simulink library "sm_boom_lift_crawler_lib"  (R2026a)
settings: Solver=VariableStepAuto
undefined symbols (not defined in the file): B, b, base_clr_a, base_clr_d, base_clr_e, base_clr_h, base_clr_s, base_h, base_opc, base_rho, base_t, base_w, F, lines, motion, overlap_l, valves, X, Y, Z
libraries: nesl_utility x155, fl_lib x72, sm_lib x38, SimscapeFluids_lib x18, $bdroot x2, simulink_extras x1, simulink x1, Custom_Valves x1
(part 1 of 4)
Description:
  | Copyright 2020-2026 The MathWorks, Inc.
settings Model: Creator=smiller  LastModifiedBy=smiller

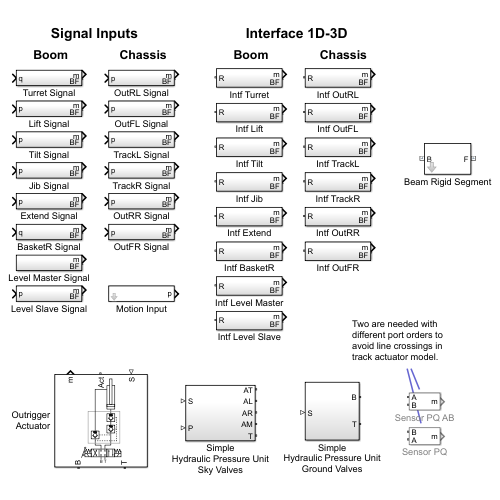
[thumbnail: Simulink's stored preview of the top-level diagram]
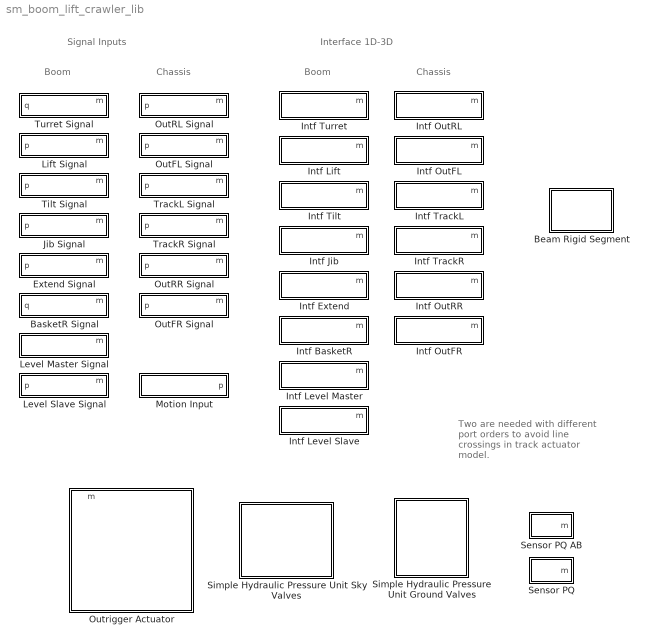
== system sm_boom_lift_crawler_lib ==
  note: Two are needed with different port orders to avoid line crossings in track actuator model.
  note: Boom
  note: Interface 1D-3D
  note: Chassis
  note: Boom
  note: Signal Inputs
  note: Chassis
  BasketR Signal : Subsystem
  Beam Rigid Segment : Subsystem  mask{beam_h=base_h, beam_w=base_w, beam_t=base_t, beam_l=overlap_l, beam_rho=base_rho, clr_d=base_clr_d, clr_s=base_clr_s, clr_a=base_clr_a, clr_e=base_clr_e, clr_h=base_clr_h, opc=base_opc}
      mask prompts: beam_h "Height (ft)"; beam_w "Width (ft)"; beam_t "Thickness (ft)"; beam_l "Length (ft)"; beam_rho "Density (kg/m^3)"; clr_d "Diffuse Color"; clr_s "Specular Color"; clr_a "Ambient Color"; clr_e "Emissive Color"; clr_h "Shininess"; opc "Opacity (0-1)"
      mask init:
      | beam_extr = [...
      |      beam_w/2  beam_h/2;
      |     -beam_w/2  beam_h/2;
      |     -beam_w/2 -beam_h/2;
      |      beam_w/2 -beam_h/2;
      |      beam_w/2  beam_h/2;
      |      (beam_w/2-beam_t)  (beam_h/2-beam_t);
      |      (beam_w/2-beam_t) -(beam_h/2-beam_t);
      |     -(beam_w/2-beam_t) -(beam_h/2-beam_t);
      |     -(beam_w/2-beam_t)  (beam_h/2-beam_t);
      |      (beam_w/2-beam_t)  (beam_h/2-beam_t);
      |     ];
      mask DialogControl cont_vis Prompt: Visualization
  Extend Signal : Subsystem
  Intf BasketR : Subsystem
  Intf Extend : Subsystem
  Intf Jib : Subsystem
  Intf Level Master : Subsystem
  Intf Level Slave : Subsystem
  Intf Lift : Subsystem
  Intf OutFL : Subsystem
  Intf OutFR : Subsystem
  Intf OutRL : Subsystem
  Intf OutRR : Subsystem
  Intf Tilt : Subsystem
  Intf TrackL : Subsystem
  Intf TrackR : Subsystem
  Intf Turret : Subsystem
  Jib Signal : Subsystem
  Level Master Signal : Subsystem
  Level Slave Signal : Subsystem
  Lift Signal : Subsystem
  Motion Input : Subsystem  mask{vec_t=motion.turret.t, vec_q=motion.turret.q}
      mask prompts: vec_t "Time"; vec_q "Angles (rad)"
  OutFL Signal : Subsystem
  OutFR Signal : Subsystem
  OutRL Signal : Subsystem
  OutRR Signal : Subsystem
  Outrigger Actuator : Subsystem
      mask Display: image('sh009.svg')
  Sensor PQ : Subsystem
  Sensor PQ AB : Subsystem
  Simple Hydraulic Pressure Unit Ground Valves : Subsystem
  Simple Hydraulic Pressure Unit Sky Valves : Subsystem
  Tilt Signal : Subsystem
  TrackL Signal : Subsystem
  TrackR Signal : Subsystem
  Turret Signal : Subsystem

== system sm_boom_lift_crawler_lib/BasketR Signal ==
  q : Inport
  Bus Creator1 : BusCreator  Inputs=3
  PS-Simulink Converter1 : nesl_utility/PS-Simulink Converter  PhysicalDomain=network_engine_domain  SubClassName=ps_output  LeftPortType=input  RightPortType=output  PseudoPeriodic=off  Frequencies=[]  VectorFormat=1-D array  Unit=inherit  AffineConversion=off
  PS-Simulink Converter2 : nesl_utility/PS-Simulink Converter  PhysicalDomain=network_engine_domain  SubClassName=ps_output  LeftPortType=input  RightPortType=output  PseudoPeriodic=off  Frequencies=[]  VectorFormat=1-D array  Unit=inherit  AffineConversion=off
  PS-Simulink Converter3 : nesl_utility/PS-Simulink Converter  PhysicalDomain=network_engine_domain  SubClassName=ps_output  LeftPortType=input  RightPortType=output  PseudoPeriodic=off  Frequencies=[]  VectorFormat=1-D array  Unit=inherit  AffineConversion=off
  Revolute BasketR : sm_lib/Joints/Revolute Joint  JointMode=Normal  CompositeWrenchDir=FollowerOnBase  CompositeWrenchFrame=BaseFrame  SenseConstraintForce=off  SenseConstraintTorque=off  SenseTotalForce=off  SenseTotalTorque=off  PositionTargetSpecify=on  PositionTargetPriority=High  PositionTargetValue=0  PositionTargetValueUnits=deg  VelocityTargetSpecify=off  VelocityTargetPriority=High  VelocityTargetValue=0  VelocityTargetValueUnits=deg/s  EquilibriumPosition=0  EquilibriumPositionUnits=rad  SpringStiffness=0  SpringStiffnessUnits=N*m/rad  DampingCoefficient=b.r.joint  DampingCoefficientUnits=N*m/(rad/s)  LowerLimitSpecify=on  LowerLimitBound=-180  LowerLimitBoundUnits=deg  LowerLimitStiffness=1e4  LowerLimitStiffnessUnits=N*m/deg  LowerLimitDamping=10  LowerLimitDampingUnits=N*m/(deg/s)  LowerLimitTransitionRegionWidth=0.1  LowerLimitTransitionRegionWidthUnits=deg  UpperLimitSpecify=on  UpperLimitBound=180  UpperLimitBoundUnits=deg  UpperLimitStiffness=1e4  UpperLimitStiffnessUnits=N*m/deg  UpperLimitDamping=10  UpperLimitDampingUnits=N*m/(deg/s)  UpperLimitTransitionRegionWidth=0.1  UpperLimitTransitionRegionWidthUnits=deg  TorqueActuationMode=ComputedTorque  MotionActuationMode=InputMotion  SensePosition=on  SenseVelocity=on  SenseAcceleration=off  SenseTorqueForce=on  SenseLowerLimitTorqueForce=off  SenseUpperLimitTorqueForce=off
  Simscape Bus3 : SimscapeBus  HierarchyStrings=B;F
  Simulink-PS Converter : nesl_utility/Simulink-PS Converter  PhysicalDomain=network_engine_domain  SubClassName=ps_input  LeftPortType=input  RightPortType=output  PseudoPeriodic=off  Frequencies=[]  NoiseDistribution=none  NoiseParameters=[]  Unit=rad  AffineConversion=off  FilteringAndDerivatives=filter  SimscapeFilterOrder=2  InputFilterTimeConstant=0.1  UdotUserProvided=0
  BF : PMIOPort  Side=Right
  m : Outport
  wires:
  PS-Simulink Converter3/1 -> Bus Creator1/3  "t"
  PS-Simulink Converter1/1 -> Bus Creator1/1  "q"
  PS-Simulink Converter2/1 -> Bus Creator1/2  "w"
  Bus Creator1/1 -> m/1  "BasketR"
  q/1 -> Simulink-PS Converter/1
  connections:
  PS-Simulink Converter3/LConn1 -- Revolute BasketR/RConn4
  Revolute BasketR/LConn2 -- Simulink-PS Converter/RConn1
  Simscape Bus3/LConn1 -- Revolute BasketR/LConn1
  Revolute BasketR/RConn3 -- PS-Simulink Converter2/LConn1
  Simscape Bus3/LConn2 -- Revolute BasketR/RConn1
  PS-Simulink Converter1/LConn1 -- Revolute BasketR/RConn2
  Simscape Bus3/RConn1 -- BF/RConn1

== system sm_boom_lift_crawler_lib/Beam Rigid Segment ==
  Bottom : sm_lib/Body Elements/Brick Solid  BrickDimensions=[beam_w beam_t overlap_l]  BrickDimensionsUnits=ft  ExportEntireGeometry=off  InertiaType=CalculateFromGeometry  BasedOnType=Density  Density=beam_rho  DensityUnits=kg/m^3  Mass=1  MassUnits=kg  CenterOfMass=[0 0 0]  CenterOfMassUnits=m  MomentsOfInertia=[1 1 1]  MomentsOfInertiaUnits=kg*m^2  ProductsOfInertia=[0 0 0]  ProductsOfInertiaUnits=kg*m^2  GraphicType=FromGeometry  MarkerShape=Sphere  MarkerSize=10  GraphicVisPropType=SimpleVisualProperties  GraphicDiffuseColor=clr_d  GraphicOpacity=opc  GraphicSpecularColor=clr_s  GraphicAmbientColor=clr_a  GraphicEmissiveColor=clr_e  GraphicShininess=clr_h  DoExposeReferenceFrame=on  SerializedFrames=<Frames/>
  Left : sm_lib/Body Elements/Brick Solid  BrickDimensions=[beam_t beam_h-beam_t*2 overlap_l]  BrickDimensionsUnits=ft  ExportEntireGeometry=off  InertiaType=CalculateFromGeometry  BasedOnType=Density  Density=beam_rho  DensityUnits=kg/m^3  Mass=1  MassUnits=kg  CenterOfMass=[0 0 0]  CenterOfMassUnits=m  MomentsOfInertia=[1 1 1]  MomentsOfInertiaUnits=kg*m^2  ProductsOfInertia=[0 0 0]  ProductsOfInertiaUnits=kg*m^2  GraphicType=FromGeometry  MarkerShape=Sphere  MarkerSize=10  GraphicVisPropType=SimpleVisualProperties  GraphicDiffuseColor=clr_d  GraphicOpacity=opc  GraphicSpecularColor=clr_s  GraphicAmbientColor=clr_a  GraphicEmissiveColor=clr_e  GraphicShininess=clr_h  DoExposeReferenceFrame=on  SerializedFrames=<Frames/>
  Right : sm_lib/Body Elements/Brick Solid  BrickDimensions=[beam_t beam_h-beam_t*2 overlap_l]  BrickDimensionsUnits=ft  ExportEntireGeometry=off  InertiaType=CalculateFromGeometry  BasedOnType=Density  Density=beam_rho  DensityUnits=kg/m^3  Mass=1  MassUnits=kg  CenterOfMass=[0 0 0]  CenterOfMassUnits=m  MomentsOfInertia=[1 1 1]  MomentsOfInertiaUnits=kg*m^2  ProductsOfInertia=[0 0 0]  ProductsOfInertiaUnits=kg*m^2  GraphicType=FromGeometry  MarkerShape=Sphere  MarkerSize=10  GraphicVisPropType=SimpleVisualProperties  GraphicDiffuseColor=clr_d  GraphicOpacity=opc  GraphicSpecularColor=clr_s  GraphicAmbientColor=clr_a  GraphicEmissiveColor=clr_e  GraphicShininess=clr_h  DoExposeReferenceFrame=on  SerializedFrames=<Frames/>
  Top : sm_lib/Body Elements/Brick Solid  BrickDimensions=[beam_w beam_t overlap_l]  BrickDimensionsUnits=ft  ExportEntireGeometry=off  InertiaType=CalculateFromGeometry  BasedOnType=Density  Density=beam_rho  DensityUnits=kg/m^3  Mass=1  MassUnits=kg  CenterOfMass=[0 0 0]  CenterOfMassUnits=m  MomentsOfInertia=[1 1 1]  MomentsOfInertiaUnits=kg*m^2  ProductsOfInertia=[0 0 0]  ProductsOfInertiaUnits=kg*m^2  GraphicType=FromGeometry  MarkerShape=Sphere  MarkerSize=10  GraphicVisPropType=SimpleVisualProperties  GraphicDiffuseColor=clr_d  GraphicOpacity=opc  GraphicSpecularColor=clr_s  GraphicAmbientColor=clr_a  GraphicEmissiveColor=clr_e  GraphicShininess=clr_h  DoExposeReferenceFrame=on  SerializedFrames=<Frames/>
  Transform B Center : sm_lib/Frames and Transforms/Rigid Transform  RotationMethod=None  FollAlignAxisA=+X  BaseAlignAxisA=+Y  FollAlignAxisB=+Y  BaseAlignAxisB=+Z  RotationStandardAxis=+Z  RotationAngle=0.0  RotationAngleUnits=deg  RotationArbitraryAxis=[0 0 1]  RotationSequenceAxes=FollowerAxes  RotationSequence=XYX  RotationSequenceAngles=[0 0 0]  RotationSequenceAnglesUnits=deg  RotationMatrix=[1 0 0; 0 1 0; 0 0 1]  Quaternion=[1 0 0 0]  TranslationMethod=StandardAxis  TranslationCartesianOffset=[0 0 0]  TranslationCartesianOffsetUnits=ft  TranslationStandardAxis=+Z  TranslationStandardOffset=overlap_l/2  TranslationStandardOffsetUnits=ft  TranslationROffset=0  TranslationROffsetUnits=m  TranslationThetaOffset=0  TranslationThetaOffsetUnits=deg  TranslationZOffset=0  TranslationZOffsetUnits=m
  Transform Bottom : sm_lib/Frames and Transforms/Rigid Transform  RotationMethod=None  FollAlignAxisA=+X  BaseAlignAxisA=+Y  FollAlignAxisB=+Y  BaseAlignAxisB=+Z  RotationStandardAxis=+Y  RotationAngle=0.0  RotationAngleUnits=deg  RotationArbitraryAxis=[0 0 1]  RotationSequenceAxes=FollowerAxes  RotationSequence=XYX  RotationSequenceAngles=[0 0 0]  RotationSequenceAnglesUnits=deg  RotationMatrix=[1 0 0; 0 1 0; 0 0 1]  Quaternion=[1 0 0 0]  TranslationMethod=StandardAxis  TranslationCartesianOffset=[0 0 0]  TranslationCartesianOffsetUnits=ft  TranslationStandardAxis=+Y  TranslationStandardOffset=(beam_h-beam_t)/2  TranslationStandardOffsetUnits=ft  TranslationROffset=0  TranslationROffsetUnits=m  TranslationThetaOffset=0  TranslationThetaOffsetUnits=deg  TranslationZOffset=0  TranslationZOffsetUnits=m
  Transform Center F : sm_lib/Frames and Transforms/Rigid Transform  RotationMethod=None  FollAlignAxisA=+X  BaseAlignAxisA=+Y  FollAlignAxisB=+Y  BaseAlignAxisB=+Z  RotationStandardAxis=+Z  RotationAngle=0.0  RotationAngleUnits=deg  RotationArbitraryAxis=[0 0 1]  RotationSequenceAxes=FollowerAxes  RotationSequence=XYX  RotationSequenceAngles=[0 0 0]  RotationSequenceAnglesUnits=deg  RotationMatrix=[1 0 0; 0 1 0; 0 0 1]  Quaternion=[1 0 0 0]  TranslationMethod=StandardAxis  TranslationCartesianOffset=[0 0 0]  TranslationCartesianOffsetUnits=ft  TranslationStandardAxis=+Z  TranslationStandardOffset=overlap_l/2  TranslationStandardOffsetUnits=ft  TranslationROffset=0  TranslationROffsetUnits=m  TranslationThetaOffset=0  TranslationThetaOffsetUnits=deg  TranslationZOffset=0  TranslationZOffsetUnits=m
  Transform Left : sm_lib/Frames and Transforms/Rigid Transform  RotationMethod=None  FollAlignAxisA=+X  BaseAlignAxisA=+Y  FollAlignAxisB=+Y  BaseAlignAxisB=+Z  RotationStandardAxis=+Y  RotationAngle=0.0  RotationAngleUnits=deg  RotationArbitraryAxis=[0 0 1]  RotationSequenceAxes=FollowerAxes  RotationSequence=XYX  RotationSequenceAngles=[0 0 0]  RotationSequenceAnglesUnits=deg  RotationMatrix=[1 0 0; 0 1 0; 0 0 1]  Quaternion=[1 0 0 0]  TranslationMethod=StandardAxis  TranslationCartesianOffset=[0 0 0]  TranslationCartesianOffsetUnits=ft  TranslationStandardAxis=+X  TranslationStandardOffset=(beam_w-beam_t)/2  TranslationStandardOffsetUnits=ft  TranslationROffset=0  TranslationROffsetUnits=m  TranslationThetaOffset=0  TranslationThetaOffsetUnits=deg  TranslationZOffset=0  TranslationZOffsetUnits=m
  Transform Right : sm_lib/Frames and Transforms/Rigid Transform  RotationMethod=None  FollAlignAxisA=+X  BaseAlignAxisA=+Y  FollAlignAxisB=+Y  BaseAlignAxisB=+Z  RotationStandardAxis=+Y  RotationAngle=0.0  RotationAngleUnits=deg  RotationArbitraryAxis=[0 0 1]  RotationSequenceAxes=FollowerAxes  RotationSequence=XYX  RotationSequenceAngles=[0 0 0]  RotationSequenceAnglesUnits=deg  RotationMatrix=[1 0 0; 0 1 0; 0 0 1]  Quaternion=[1 0 0 0]  TranslationMethod=StandardAxis  TranslationCartesianOffset=[0 0 0]  TranslationCartesianOffsetUnits=ft  TranslationStandardAxis=+X  TranslationStandardOffset=(beam_w-beam_t)/2  TranslationStandardOffsetUnits=ft  TranslationROffset=0  TranslationROffsetUnits=m  TranslationThetaOffset=0  TranslationThetaOffsetUnits=deg  TranslationZOffset=0  TranslationZOffsetUnits=m
  Transform Top : sm_lib/Frames and Transforms/Rigid Transform  RotationMethod=None  FollAlignAxisA=+X  BaseAlignAxisA=+Y  FollAlignAxisB=+Y  BaseAlignAxisB=+Z  RotationStandardAxis=+Y  RotationAngle=0.0  RotationAngleUnits=deg  RotationArbitraryAxis=[0 0 1]  RotationSequenceAxes=FollowerAxes  RotationSequence=XYX  RotationSequenceAngles=[0 0 0]  RotationSequenceAnglesUnits=deg  RotationMatrix=[1 0 0; 0 1 0; 0 0 1]  Quaternion=[1 0 0 0]  TranslationMethod=StandardAxis  TranslationCartesianOffset=[0 0 0]  TranslationCartesianOffsetUnits=ft  TranslationStandardAxis=+Y  TranslationStandardOffset=(beam_h-beam_t)/2  TranslationStandardOffsetUnits=ft  TranslationROffset=0  TranslationROffsetUnits=m  TranslationThetaOffset=0  TranslationThetaOffsetUnits=deg  TranslationZOffset=0  TranslationZOffsetUnits=m
  B : PMIOPort  Side=Left
  F : PMIOPort  Port=2  Side=Right
  connections:
  Left/RConn1 -- Transform Left/LConn1
  Right/RConn1 -- Transform Right/RConn1
  Bottom/RConn1 -- Transform Bottom/LConn1
  Top/RConn1 -- Transform Top/RConn1
  Transform Left/RConn1 -- Transform Top/LConn1 -- Transform Right/LConn1 -- Transform B Center/RConn1 -- Transform Center F/LConn1 -- Transform Bottom/RConn1
  Transform Center F/RConn1 -- F/RConn1
  Transform B Center/LConn1 -- B/RConn1

== system sm_boom_lift_crawler_lib/Extend Signal ==
  p : Inport
  Bus Creator1 : BusCreator  Inputs=3
  PS-Simulink Converter1 : nesl_utility/PS-Simulink Converter  PhysicalDomain=network_engine_domain  SubClassName=ps_output  LeftPortType=input  RightPortType=output  PseudoPeriodic=off  Frequencies=[]  VectorFormat=1-D array  Unit=inherit  AffineConversion=off
  PS-Simulink Converter2 : nesl_utility/PS-Simulink Converter  PhysicalDomain=network_engine_domain  SubClassName=ps_output  LeftPortType=input  RightPortType=output  PseudoPeriodic=off  Frequencies=[]  VectorFormat=1-D array  Unit=inherit  AffineConversion=off
  PS-Simulink Converter3 : nesl_utility/PS-Simulink Converter  PhysicalDomain=network_engine_domain  SubClassName=ps_output  LeftPortType=input  RightPortType=output  PseudoPeriodic=off  Frequencies=[]  VectorFormat=1-D array  Unit=inherit  AffineConversion=off
  Prismatic Extend : sm_lib/Joints/Prismatic Joint  JointMode=Normal  CompositeWrenchDir=FollowerOnBase  CompositeWrenchFrame=BaseFrame  SenseConstraintForce=off  SenseConstraintTorque=off  SenseTotalForce=off  SenseTotalTorque=off  PositionTargetSpecify=on  PositionTargetPriority=High  PositionTargetValue=pz0.stickboom.extend  PositionTargetValueUnits=in  VelocityTargetSpecify=off  VelocityTargetPriority=High  VelocityTargetValue=0  VelocityTargetValueUnits=m/s  EquilibriumPosition=0  EquilibriumPositionUnits=m  SpringStiffness=0  SpringStiffnessUnits=N/m  DampingCoefficient=0  DampingCoefficientUnits=N/(m/s)  LowerLimitSpecify=off  LowerLimitBound=0.125  LowerLimitBoundUnits=in  LowerLimitStiffness=1e6  LowerLimitStiffnessUnits=N/m  LowerLimitDamping=1e3  LowerLimitDampingUnits=N/(m/s)  LowerLimitTransitionRegionWidth=1e-4  LowerLimitTransitionRegionWidthUnits=m  UpperLimitSpecify=off  UpperLimitBound=170  UpperLimitBoundUnits=in  UpperLimitStiffness=1e6  UpperLimitStiffnessUnits=N/m  UpperLimitDamping=1e3  UpperLimitDampingUnits=N/(m/s)  UpperLimitTransitionRegionWidth=1e-4  UpperLimitTransitionRegionWidthUnits=m  TorqueActuationMode=ComputedTorque  MotionActuationMode=InputMotion  SensePosition=on  SenseVelocity=on  SenseAcceleration=off  SenseTorqueForce=on  SenseLowerLimitTorqueForce=off  SenseUpperLimitTorqueForce=off
  Simscape Bus3 : SimscapeBus  HierarchyStrings=B;F
  Simulink-PS Converter : nesl_utility/Simulink-PS Converter  PhysicalDomain=network_engine_domain  SubClassName=ps_input  LeftPortType=input  RightPortType=output  PseudoPeriodic=off  Frequencies=[]  NoiseDistribution=none  NoiseParameters=[]  Unit=m  AffineConversion=off  FilteringAndDerivatives=filter  SimscapeFilterOrder=2  InputFilterTimeConstant=0.2  UdotUserProvided=0
  BF : PMIOPort  Side=Right
  m : Outport
  wires:
  PS-Simulink Converter3/1 -> Bus Creator1/3  "f"
  Bus Creator1/1 -> m/1  "Extend"
  PS-Simulink Converter2/1 -> Bus Creator1/2  "v"
  p/1 -> Simulink-PS Converter/1
  PS-Simulink Converter1/1 -> Bus Creator1/1  "p"
  connections:
  PS-Simulink Converter3/LConn1 -- Prismatic Extend/RConn4
  PS-Simulink Converter2/LConn1 -- Prismatic Extend/RConn3
  Prismatic Extend/LConn2 -- Simulink-PS Converter/RConn1
  BF/RConn1 -- Simscape Bus3/RConn1
  Simscape Bus3/LConn1 -- Prismatic Extend/LConn1
  Prismatic Extend/RConn1 -- Simscape Bus3/LConn2
  PS-Simulink Converter1/LConn1 -- Prismatic Extend/RConn2

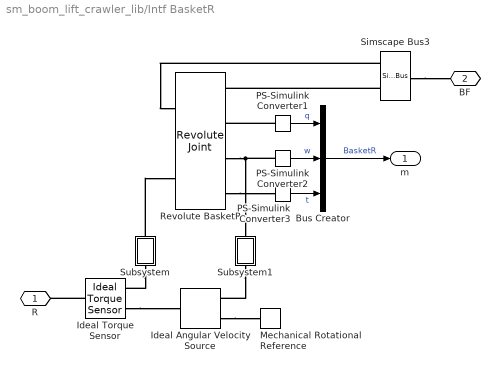
== system sm_boom_lift_crawler_lib/Intf BasketR ==
  Bus Creator : BusCreator  Inputs=3
  Ideal Angular Velocity Source : fl_lib/Mechanical/Mechanical Sources/Ideal Angular Velocity Source
  Ideal Torque Sensor : fl_lib/Mechanical/Mechanical Sensors/Ideal Torque Sensor
  Mechanical Rotational Reference : fl_lib/Mechanical/Rotational Elements/Mechanical Rotational Reference
  PS-Simulink Converter1 : nesl_utility/PS-Simulink Converter  PhysicalDomain=network_engine_domain  SubClassName=ps_output  LeftPortType=input  RightPortType=output  PseudoPeriodic=off  Frequencies=[]  VectorFormat=1-D array  Unit=inherit  AffineConversion=off
  PS-Simulink Converter2 : nesl_utility/PS-Simulink Converter  PhysicalDomain=network_engine_domain  SubClassName=ps_output  LeftPortType=input  RightPortType=output  PseudoPeriodic=off  Frequencies=[]  VectorFormat=1-D array  Unit=inherit  AffineConversion=off
  PS-Simulink Converter3 : nesl_utility/PS-Simulink Converter  PhysicalDomain=network_engine_domain  SubClassName=ps_output  LeftPortType=input  RightPortType=output  PseudoPeriodic=off  Frequencies=[]  VectorFormat=1-D array  Unit=inherit  AffineConversion=off
  Revolute BasketR : sm_lib/Joints/Revolute Joint  JointMode=Normal  CompositeWrenchDir=FollowerOnBase  CompositeWrenchFrame=BaseFrame  SenseConstraintForce=off  SenseConstraintTorque=off  SenseTotalForce=off  SenseTotalTorque=off  PositionTargetSpecify=on  PositionTargetPriority=High  PositionTargetValue=0  PositionTargetValueUnits=deg  VelocityTargetSpecify=off  VelocityTargetPriority=High  VelocityTargetValue=0  VelocityTargetValueUnits=deg/s  EquilibriumPosition=0  EquilibriumPositionUnits=rad  SpringStiffness=0  SpringStiffnessUnits=N*m/rad  DampingCoefficient=b.r.joint  DampingCoefficientUnits=N*m/(rad/s)  LowerLimitSpecify=on  LowerLimitBound=-180  LowerLimitBoundUnits=deg  LowerLimitStiffness=1e4  LowerLimitStiffnessUnits=N*m/deg  LowerLimitDamping=10  LowerLimitDampingUnits=N*m/(deg/s)  LowerLimitTransitionRegionWidth=0.1  LowerLimitTransitionRegionWidthUnits=deg  UpperLimitSpecify=on  UpperLimitBound=180  UpperLimitBoundUnits=deg  UpperLimitStiffness=1e4  UpperLimitStiffnessUnits=N*m/deg  UpperLimitDamping=10  UpperLimitDampingUnits=N*m/(deg/s)  UpperLimitTransitionRegionWidth=0.1  UpperLimitTransitionRegionWidthUnits=deg  TorqueActuationMode=InputTorque  MotionActuationMode=ComputedMotion  SensePosition=on  SenseVelocity=on  SenseAcceleration=off  SenseTorqueForce=on  SenseLowerLimitTorqueForce=off  SenseUpperLimitTorqueForce=off
  Simscape Bus3 : SimscapeBus  HierarchyStrings=B;F
  Subsystem : Subsystem
  Subsystem1 : Subsystem
  R : PMIOPort  Side=Left
  BF : PMIOPort  Port=2  Side=Right
  m : Outport
  wires:
  PS-Simulink Converter1/1 -> Bus Creator/1  "q"
  Bus Creator/1 -> m/1  "BasketR"
  PS-Simulink Converter2/1 -> Bus Creator/2  "w"
  PS-Simulink Converter3/1 -> Bus Creator/3  "t"
  connections:
  Simscape Bus3/LConn1 -- Revolute BasketR/LConn1
  Revolute BasketR/RConn3 -- Subsystem1/LConn1 -- PS-Simulink Converter2/LConn1
  Subsystem/RConn1 -- Revolute BasketR/LConn2
  Ideal Torque Sensor/LConn1 -- R/RConn1
  Simscape Bus3/LConn2 -- Revolute BasketR/RConn1
  PS-Simulink Converter1/LConn1 -- Revolute BasketR/RConn2
  Simscape Bus3/RConn1 -- BF/RConn1
  Subsystem1/RConn1 -- Ideal Angular Velocity Source/RConn1
  Ideal Angular Velocity Source/RConn2 -- Mechanical Rotational Reference/LConn1
  Ideal Torque Sensor/RConn1 -- Ideal Angular Velocity Source/LConn1
  Subsystem/LConn1 -- Ideal Torque Sensor/RConn2
  Revolute BasketR/RConn4 -- PS-Simulink Converter3/LConn1

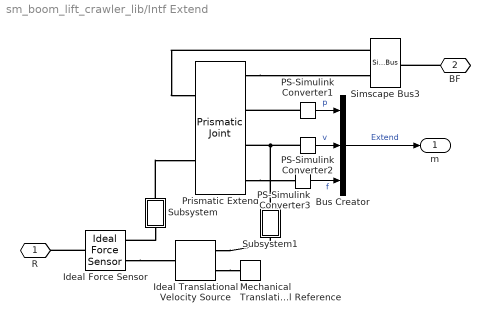
== system sm_boom_lift_crawler_lib/Intf Extend ==
  Bus Creator : BusCreator  Inputs=3
  Ideal Force Sensor : fl_lib/Mechanical/Mechanical Sensors/Ideal Force Sensor
  Ideal Translational Velocity Source : fl_lib/Mechanical/Mechanical Sources/Ideal Translational Velocity Source
  Mechanical Translational Reference : fl_lib/Mechanical/Translational Elements/Mechanical Translational Reference
  PS-Simulink Converter1 : nesl_utility/PS-Simulink Converter  PhysicalDomain=network_engine_domain  SubClassName=ps_output  LeftPortType=input  RightPortType=output  PseudoPeriodic=off  Frequencies=[]  VectorFormat=1-D array  Unit=inherit  AffineConversion=off
  PS-Simulink Converter2 : nesl_utility/PS-Simulink Converter  PhysicalDomain=network_engine_domain  SubClassName=ps_output  LeftPortType=input  RightPortType=output  PseudoPeriodic=off  Frequencies=[]  VectorFormat=1-D array  Unit=inherit  AffineConversion=off
  PS-Simulink Converter3 : nesl_utility/PS-Simulink Converter  PhysicalDomain=network_engine_domain  SubClassName=ps_output  LeftPortType=input  RightPortType=output  PseudoPeriodic=off  Frequencies=[]  VectorFormat=1-D array  Unit=inherit  AffineConversion=off
  Prismatic Extend : sm_lib/Joints/Prismatic Joint  JointMode=Normal  CompositeWrenchDir=FollowerOnBase  CompositeWrenchFrame=BaseFrame  SenseConstraintForce=off  SenseConstraintTorque=off  SenseTotalForce=off  SenseTotalTorque=off  PositionTargetSpecify=on  PositionTargetPriority=High  PositionTargetValue=pz0.stickboom.extend  PositionTargetValueUnits=in  VelocityTargetSpecify=off  VelocityTargetPriority=High  VelocityTargetValue=0  VelocityTargetValueUnits=m/s  EquilibriumPosition=0  EquilibriumPositionUnits=m  SpringStiffness=0  SpringStiffnessUnits=N/m  DampingCoefficient=0  DampingCoefficientUnits=N/(m/s)  LowerLimitSpecify=off  LowerLimitBound=0.125  LowerLimitBoundUnits=in  LowerLimitStiffness=1e6  LowerLimitStiffnessUnits=N/m  LowerLimitDamping=1e3  LowerLimitDampingUnits=N/(m/s)  LowerLimitTransitionRegionWidth=1e-4  LowerLimitTransitionRegionWidthUnits=m  UpperLimitSpecify=off  UpperLimitBound=170  UpperLimitBoundUnits=in  UpperLimitStiffness=1e6  UpperLimitStiffnessUnits=N/m  UpperLimitDamping=1e3  UpperLimitDampingUnits=N/(m/s)  UpperLimitTransitionRegionWidth=1e-4  UpperLimitTransitionRegionWidthUnits=m  TorqueActuationMode=InputTorque  MotionActuationMode=ComputedMotion  SensePosition=on  SenseVelocity=on  SenseAcceleration=off  SenseTorqueForce=on  SenseLowerLimitTorqueForce=off  SenseUpperLimitTorqueForce=off
  Simscape Bus3 : SimscapeBus  HierarchyStrings=B;F
  Subsystem : Subsystem
  Subsystem1 : Subsystem
  R : PMIOPort  Side=Left
  BF : PMIOPort  Port=2  Side=Right
  m : Outport
  wires:
  PS-Simulink Converter1/1 -> Bus Creator/1  "p"
  Bus Creator/1 -> m/1  "Extend"
  PS-Simulink Converter2/1 -> Bus Creator/2  "v"
  PS-Simulink Converter3/1 -> Bus Creator/3  "f"
  connections:
  Subsystem/RConn1 -- Prismatic Extend/LConn2
  PS-Simulink Converter2/LConn1 -- Prismatic Extend/RConn3 -- Subsystem1/LConn1
  BF/RConn1 -- Simscape Bus3/RConn1
  Ideal Translational Velocity Source/RConn1 -- Subsystem1/RConn1
  Simscape Bus3/LConn1 -- Prismatic Extend/LConn1
  Prismatic Extend/RConn1 -- Simscape Bus3/LConn2
  PS-Simulink Converter1/LConn1 -- Prismatic Extend/RConn2
  Ideal Force Sensor/LConn1 -- R/RConn1
  Ideal Translational Velocity Source/RConn2 -- Mechanical Translational Reference/LConn1
  Ideal Force Sensor/RConn1 -- Ideal Translational Velocity Source/LConn1
  Subsystem/LConn1 -- Ideal Force Sensor/RConn2
  Prismatic Extend/RConn4 -- PS-Simulink Converter3/LConn1

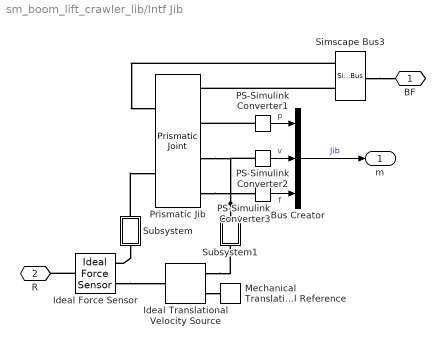
== system sm_boom_lift_crawler_lib/Intf Jib ==
  Bus Creator : BusCreator  Inputs=3
  Ideal Force Sensor : fl_lib/Mechanical/Mechanical Sensors/Ideal Force Sensor
  Ideal Translational Velocity Source : fl_lib/Mechanical/Mechanical Sources/Ideal Translational Velocity Source
  Mechanical Translational Reference : fl_lib/Mechanical/Translational Elements/Mechanical Translational Reference
  PS-Simulink Converter1 : nesl_utility/PS-Simulink Converter  PhysicalDomain=network_engine_domain  SubClassName=ps_output  LeftPortType=input  RightPortType=output  PseudoPeriodic=off  Frequencies=[]  VectorFormat=1-D array  Unit=inherit  AffineConversion=off
  PS-Simulink Converter2 : nesl_utility/PS-Simulink Converter  PhysicalDomain=network_engine_domain  SubClassName=ps_output  LeftPortType=input  RightPortType=output  PseudoPeriodic=off  Frequencies=[]  VectorFormat=1-D array  Unit=inherit  AffineConversion=off
  PS-Simulink Converter3 : nesl_utility/PS-Simulink Converter  PhysicalDomain=network_engine_domain  SubClassName=ps_output  LeftPortType=input  RightPortType=output  PseudoPeriodic=off  Frequencies=[]  VectorFormat=1-D array  Unit=inherit  AffineConversion=off
  Prismatic Jib : sm_lib/Joints/Prismatic Joint  JointMode=Normal  CompositeWrenchDir=FollowerOnBase  CompositeWrenchFrame=BaseFrame  SenseConstraintForce=off  SenseConstraintTorque=off  SenseTotalForce=off  SenseTotalTorque=off  PositionTargetSpecify=on  PositionTargetPriority=High  PositionTargetValue=0  PositionTargetValueUnits=in  VelocityTargetSpecify=off  VelocityTargetPriority=High  VelocityTargetValue=0  VelocityTargetValueUnits=m/s  EquilibriumPosition=0  EquilibriumPositionUnits=m  SpringStiffness=0  SpringStiffnessUnits=N/m  DampingCoefficient=100  DampingCoefficientUnits=N/(m/s)  LowerLimitSpecify=off  LowerLimitBound=0.925  LowerLimitBoundUnits=in  LowerLimitStiffness=1e6  LowerLimitStiffnessUnits=N/m  LowerLimitDamping=1e3  LowerLimitDampingUnits=N/(m/s)  LowerLimitTransitionRegionWidth=1e-4  LowerLimitTransitionRegionWidthUnits=m  UpperLimitSpecify=off  UpperLimitBound=14  UpperLimitBoundUnits=in  UpperLimitStiffness=1e6  UpperLimitStiffnessUnits=N/m  UpperLimitDamping=1e3  UpperLimitDampingUnits=N/(m/s)  UpperLimitTransitionRegionWidth=1e-4  UpperLimitTransitionRegionWidthUnits=m  TorqueActuationMode=InputTorque  MotionActuationMode=ComputedMotion  SensePosition=on  SenseVelocity=on  SenseAcceleration=off  SenseTorqueForce=on  SenseLowerLimitTorqueForce=off  SenseUpperLimitTorqueForce=off
  Simscape Bus3 : SimscapeBus  HierarchyStrings=B;F
  Subsystem : Subsystem
  Subsystem1 : Subsystem
  BF : PMIOPort  Side=Right
  R : PMIOPort  Port=2  Side=Left
  m : Outport
  wires:
  PS-Simulink Converter1/1 -> Bus Creator/1  "p"
  Bus Creator/1 -> m/1  "Jib"
  PS-Simulink Converter2/1 -> Bus Creator/2  "v"
  PS-Simulink Converter3/1 -> Bus Creator/3  "f"
  connections:
  Subsystem1/LConn1 -- Prismatic Jib/RConn3 -- PS-Simulink Converter2/LConn1
  PS-Simulink Converter1/LConn1 -- Prismatic Jib/RConn2
  Simscape Bus3/LConn1 -- Prismatic Jib/LConn1
  Ideal Force Sensor/LConn1 -- R/RConn1
  Simscape Bus3/LConn2 -- Prismatic Jib/RConn1
  Ideal Translational Velocity Source/RConn1 -- Subsystem1/RConn1
  Subsystem/RConn1 -- Prismatic Jib/LConn2
  Simscape Bus3/RConn1 -- BF/RConn1
  Ideal Translational Velocity Source/RConn2 -- Mechanical Translational Reference/LConn1
  Ideal Force Sensor/RConn1 -- Ideal Translational Velocity Source/LConn1
  Subsystem/LConn1 -- Ideal Force Sensor/RConn2
  Prismatic Jib/RConn4 -- PS-Simulink Converter3/LConn1

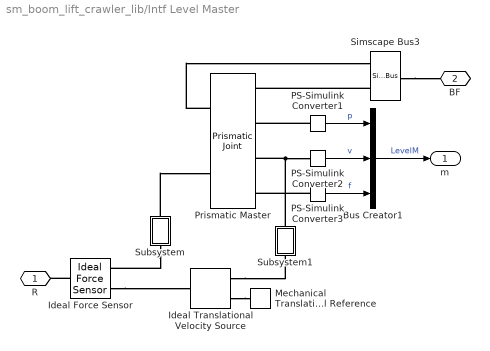
== system sm_boom_lift_crawler_lib/Intf Level Master ==
  Bus Creator1 : BusCreator  Inputs=3
  Ideal Force Sensor : fl_lib/Mechanical/Mechanical Sensors/Ideal Force Sensor
  Ideal Translational Velocity Source : fl_lib/Mechanical/Mechanical Sources/Ideal Translational Velocity Source
  Mechanical Translational Reference : fl_lib/Mechanical/Translational Elements/Mechanical Translational Reference
  PS-Simulink Converter1 : nesl_utility/PS-Simulink Converter  PhysicalDomain=network_engine_domain  SubClassName=ps_output  LeftPortType=input  RightPortType=output  PseudoPeriodic=off  Frequencies=[]  VectorFormat=1-D array  Unit=inherit  AffineConversion=off
  PS-Simulink Converter2 : nesl_utility/PS-Simulink Converter  PhysicalDomain=network_engine_domain  SubClassName=ps_output  LeftPortType=input  RightPortType=output  PseudoPeriodic=off  Frequencies=[]  VectorFormat=1-D array  Unit=inherit  AffineConversion=off
  PS-Simulink Converter3 : nesl_utility/PS-Simulink Converter  PhysicalDomain=network_engine_domain  SubClassName=ps_output  LeftPortType=input  RightPortType=output  PseudoPeriodic=off  Frequencies=[]  VectorFormat=1-D array  Unit=inherit  AffineConversion=off
  Prismatic Master : sm_lib/Joints/Prismatic Joint  JointMode=Normal  CompositeWrenchDir=FollowerOnBase  CompositeWrenchFrame=BaseFrame  SenseConstraintForce=off  SenseConstraintTorque=off  SenseTotalForce=off  SenseTotalTorque=off  PositionTargetSpecify=off  PositionTargetPriority=Low  PositionTargetValue=0  PositionTargetValueUnits=in  VelocityTargetSpecify=off  VelocityTargetPriority=High  VelocityTargetValue=0  VelocityTargetValueUnits=m/s  EquilibriumPosition=0  EquilibriumPositionUnits=m  SpringStiffness=0  SpringStiffnessUnits=N/m  DampingCoefficient=b.p.joint.i  DampingCoefficientUnits=N/(m/s)  LowerLimitSpecify=off  LowerLimitBound=-1  LowerLimitBoundUnits=m  LowerLimitStiffness=1e6  LowerLimitStiffnessUnits=N/m  LowerLimitDamping=1e3  LowerLimitDampingUnits=N/(m/s)  LowerLimitTransitionRegionWidth=1e-4  LowerLimitTransitionRegionWidthUnits=m  UpperLimitSpecify=off  UpperLimitBound=1  UpperLimitBoundUnits=m  UpperLimitStiffness=1e6  UpperLimitStiffnessUnits=N/m  UpperLimitDamping=1e3  UpperLimitDampingUnits=N/(m/s)  UpperLimitTransitionRegionWidth=1e-4  UpperLimitTransitionRegionWidthUnits=m  TorqueActuationMode=InputTorque  MotionActuationMode=ComputedMotion  SensePosition=on  SenseVelocity=on  SenseAcceleration=off  SenseTorqueForce=on  SenseLowerLimitTorqueForce=off  SenseUpperLimitTorqueForce=off
  Simscape Bus3 : SimscapeBus  HierarchyStrings=B;F
  Subsystem : Subsystem
  Subsystem1 : Subsystem
  R : PMIOPort  Side=Left
  BF : PMIOPort  Port=2  Side=Right
  m : Outport
  wires:
  PS-Simulink Converter1/1 -> Bus Creator1/1  "p"
  Bus Creator1/1 -> m/1  "LevelM"
  PS-Simulink Converter2/1 -> Bus Creator1/2  "v"
  PS-Simulink Converter3/1 -> Bus Creator1/3  "f"
  connections:
  Ideal Translational Velocity Source/RConn1 -- Subsystem1/RConn1
  Subsystem1/LConn1 -- PS-Simulink Converter2/LConn1 -- Prismatic Master/RConn3
  Prismatic Master/LConn1 -- Simscape Bus3/LConn1
  PS-Simulink Converter1/LConn1 -- Prismatic Master/RConn2
  Subsystem/RConn1 -- Prismatic Master/LConn2
  Simscape Bus3/LConn2 -- Prismatic Master/RConn1
  Simscape Bus3/RConn1 -- BF/RConn1
  Ideal Force Sensor/LConn1 -- R/RConn1
  Ideal Translational Velocity Source/RConn2 -- Mechanical Translational Reference/LConn1
  Ideal Force Sensor/RConn1 -- Ideal Translational Velocity Source/LConn1
  Subsystem/LConn1 -- Ideal Force Sensor/RConn2
  PS-Simulink Converter3/LConn1 -- Prismatic Master/RConn4

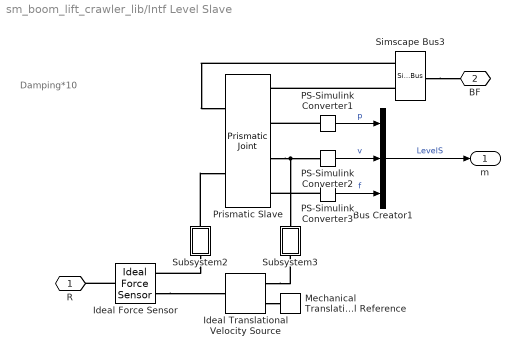
== system sm_boom_lift_crawler_lib/Intf Level Slave ==
  note: Damping*10
  Bus Creator1 : BusCreator  Inputs=3
  Ideal Force Sensor : fl_lib/Mechanical/Mechanical Sensors/Ideal Force Sensor
  Ideal Translational Velocity Source : fl_lib/Mechanical/Mechanical Sources/Ideal Translational Velocity Source
  Mechanical Translational Reference : fl_lib/Mechanical/Translational Elements/Mechanical Translational Reference
  PS-Simulink Converter1 : nesl_utility/PS-Simulink Converter  PhysicalDomain=network_engine_domain  SubClassName=ps_output  LeftPortType=input  RightPortType=output  PseudoPeriodic=off  Frequencies=[]  VectorFormat=1-D array  Unit=inherit  AffineConversion=off
  PS-Simulink Converter2 : nesl_utility/PS-Simulink Converter  PhysicalDomain=network_engine_domain  SubClassName=ps_output  LeftPortType=input  RightPortType=output  PseudoPeriodic=off  Frequencies=[]  VectorFormat=1-D array  Unit=inherit  AffineConversion=off
  PS-Simulink Converter3 : nesl_utility/PS-Simulink Converter  PhysicalDomain=network_engine_domain  SubClassName=ps_output  LeftPortType=input  RightPortType=output  PseudoPeriodic=off  Frequencies=[]  VectorFormat=1-D array  Unit=inherit  AffineConversion=off
  Prismatic Slave : sm_lib/Joints/Prismatic Joint  JointMode=Normal  CompositeWrenchDir=FollowerOnBase  CompositeWrenchFrame=BaseFrame  SenseConstraintForce=off  SenseConstraintTorque=off  SenseTotalForce=off  SenseTotalTorque=off  PositionTargetSpecify=on  PositionTargetPriority=Low  PositionTargetValue=0  PositionTargetValueUnits=in  VelocityTargetSpecify=off  VelocityTargetPriority=High  VelocityTargetValue=0  VelocityTargetValueUnits=m/s  EquilibriumPosition=0  EquilibriumPositionUnits=m  SpringStiffness=0  SpringStiffnessUnits=N/m  DampingCoefficient=b.p.joint.i*10  DampingCoefficientUnits=N/(m/s)  LowerLimitSpecify=off  LowerLimitBound=0  LowerLimitBoundUnits=in  LowerLimitStiffness=1e6  LowerLimitStiffnessUnits=N/m  LowerLimitDamping=1e3  LowerLimitDampingUnits=N/(m/s)  LowerLimitTransitionRegionWidth=1e-4  LowerLimitTransitionRegionWidthUnits=m  UpperLimitSpecify=off  UpperLimitBound=1  UpperLimitBoundUnits=in  UpperLimitStiffness=1e6  UpperLimitStiffnessUnits=N/m  UpperLimitDamping=1e3  UpperLimitDampingUnits=N/(m/s)  UpperLimitTransitionRegionWidth=1e-4  UpperLimitTransitionRegionWidthUnits=m  TorqueActuationMode=InputTorque  MotionActuationMode=ComputedMotion  SensePosition=on  SenseVelocity=on  SenseAcceleration=off  SenseTorqueForce=on  SenseLowerLimitTorqueForce=off  SenseUpperLimitTorqueForce=off
  Simscape Bus3 : SimscapeBus  HierarchyStrings=B;F
  Subsystem2 : Subsystem
  Subsystem3 : Subsystem
  R : PMIOPort  Side=Left
  BF : PMIOPort  Port=2  Side=Right
  m : Outport
  wires:
  PS-Simulink Converter1/1 -> Bus Creator1/1  "p"
  Bus Creator1/1 -> m/1  "LevelS"
  PS-Simulink Converter2/1 -> Bus Creator1/2  "v"
  PS-Simulink Converter3/1 -> Bus Creator1/3  "f"
  connections:
  Subsystem2/RConn1 -- Prismatic Slave/LConn2
  Prismatic Slave/RConn3 -- PS-Simulink Converter2/LConn1 -- Subsystem3/LConn1
  Simscape Bus3/LConn1 -- Prismatic Slave/LConn1
  PS-Simulink Converter1/LConn1 -- Prismatic Slave/RConn2
  Ideal Translational Velocity Source/RConn1 -- Subsystem3/RConn1
  Simscape Bus3/RConn1 -- BF/RConn1
  Ideal Force Sensor/LConn1 -- R/RConn1
  Simscape Bus3/LConn2 -- Prismatic Slave/RConn1
  Subsystem2/LConn1 -- Ideal Force Sensor/RConn2
  Ideal Force Sensor/RConn1 -- Ideal Translational Velocity Source/LConn1
  Ideal Translational Velocity Source/RConn2 -- Mechanical Translational Reference/LConn1
  PS-Simulink Converter3/LConn1 -- Prismatic Slave/RConn4

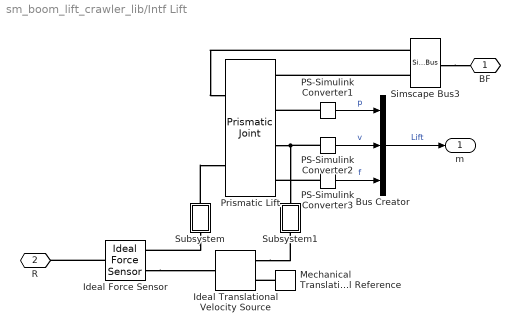
== system sm_boom_lift_crawler_lib/Intf Lift ==
  Bus Creator : BusCreator  Inputs=3
  Ideal Force Sensor : fl_lib/Mechanical/Mechanical Sensors/Ideal Force Sensor
  Ideal Translational Velocity Source : fl_lib/Mechanical/Mechanical Sources/Ideal Translational Velocity Source
  Mechanical Translational Reference : fl_lib/Mechanical/Translational Elements/Mechanical Translational Reference
  PS-Simulink Converter1 : nesl_utility/PS-Simulink Converter  PhysicalDomain=network_engine_domain  SubClassName=ps_output  LeftPortType=input  RightPortType=output  PseudoPeriodic=off  Frequencies=[]  VectorFormat=1-D array  Unit=inherit  AffineConversion=off
  PS-Simulink Converter2 : nesl_utility/PS-Simulink Converter  PhysicalDomain=network_engine_domain  SubClassName=ps_output  LeftPortType=input  RightPortType=output  PseudoPeriodic=off  Frequencies=[]  VectorFormat=1-D array  Unit=inherit  AffineConversion=off
  PS-Simulink Converter3 : nesl_utility/PS-Simulink Converter  PhysicalDomain=network_engine_domain  SubClassName=ps_output  LeftPortType=input  RightPortType=output  PseudoPeriodic=off  Frequencies=[]  VectorFormat=1-D array  Unit=inherit  AffineConversion=off
  Prismatic Lift : sm_lib/Joints/Prismatic Joint  JointMode=Normal  CompositeWrenchDir=FollowerOnBase  CompositeWrenchFrame=BaseFrame  SenseConstraintForce=off  SenseConstraintTorque=off  SenseTotalForce=off  SenseTotalTorque=off  PositionTargetSpecify=on  PositionTargetPriority=High  PositionTargetValue=0  PositionTargetValueUnits=in  VelocityTargetSpecify=off  VelocityTargetPriority=High  VelocityTargetValue=0  VelocityTargetValueUnits=m/s  EquilibriumPosition=0  EquilibriumPositionUnits=m  SpringStiffness=0  SpringStiffnessUnits=N/m  DampingCoefficient=0  DampingCoefficientUnits=N/(m/s)  LowerLimitSpecify=off  LowerLimitBound=0  LowerLimitBoundUnits=m  LowerLimitStiffness=1e6  LowerLimitStiffnessUnits=N/m  LowerLimitDamping=1e3  LowerLimitDampingUnits=N/(m/s)  LowerLimitTransitionRegionWidth=1e-4  LowerLimitTransitionRegionWidthUnits=m  UpperLimitSpecify=off  UpperLimitBound=1  UpperLimitBoundUnits=m  UpperLimitStiffness=1e6  UpperLimitStiffnessUnits=N/m  UpperLimitDamping=1e3  UpperLimitDampingUnits=N/(m/s)  UpperLimitTransitionRegionWidth=1e-4  UpperLimitTransitionRegionWidthUnits=m  TorqueActuationMode=InputTorque  MotionActuationMode=ComputedMotion  SensePosition=on  SenseVelocity=on  SenseAcceleration=off  SenseTorqueForce=on  SenseLowerLimitTorqueForce=off  SenseUpperLimitTorqueForce=off
  Simscape Bus3 : SimscapeBus  HierarchyStrings=B;F
  Subsystem : Subsystem
  Subsystem1 : Subsystem
  BF : PMIOPort  Side=Right
  R : PMIOPort  Port=2  Side=Left
  m : Outport
  wires:
  PS-Simulink Converter2/1 -> Bus Creator/2  "v"
  Bus Creator/1 -> m/1  "Lift"
  PS-Simulink Converter1/1 -> Bus Creator/1  "p"
  PS-Simulink Converter3/1 -> Bus Creator/3  "f"
  connections:
  Ideal Translational Velocity Source/RConn1 -- Subsystem1/RConn1
  Simscape Bus3/LConn2 -- Prismatic Lift/RConn1
  PS-Simulink Converter1/LConn1 -- Prismatic Lift/RConn2
  Subsystem/RConn1 -- Prismatic Lift/LConn2
  PS-Simulink Converter2/LConn1 -- Subsystem1/LConn1 -- Prismatic Lift/RConn3
  Simscape Bus3/RConn1 -- BF/RConn1
  Simscape Bus3/LConn1 -- Prismatic Lift/LConn1
  Ideal Force Sensor/LConn1 -- R/RConn1
  Mechanical Translational Reference/LConn1 -- Ideal Translational Velocity Source/RConn2
  Ideal Force Sensor/RConn1 -- Ideal Translational Velocity Source/LConn1
  Subsystem/LConn1 -- Ideal Force Sensor/RConn2
  PS-Simulink Converter3/LConn1 -- Prismatic Lift/RConn4

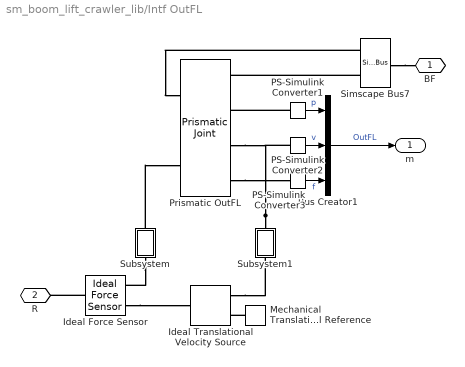
== system sm_boom_lift_crawler_lib/Intf OutFL ==
  Bus Creator1 : BusCreator  Inputs=3
  Ideal Force Sensor : fl_lib/Mechanical/Mechanical Sensors/Ideal Force Sensor
  Ideal Translational Velocity Source : fl_lib/Mechanical/Mechanical Sources/Ideal Translational Velocity Source
  Mechanical Translational Reference : fl_lib/Mechanical/Translational Elements/Mechanical Translational Reference
  PS-Simulink Converter1 : nesl_utility/PS-Simulink Converter  PhysicalDomain=network_engine_domain  SubClassName=ps_output  LeftPortType=input  RightPortType=output  PseudoPeriodic=off  Frequencies=[]  VectorFormat=1-D array  Unit=inherit  AffineConversion=off
  PS-Simulink Converter2 : nesl_utility/PS-Simulink Converter  PhysicalDomain=network_engine_domain  SubClassName=ps_output  LeftPortType=input  RightPortType=output  PseudoPeriodic=off  Frequencies=[]  VectorFormat=1-D array  Unit=inherit  AffineConversion=off
  PS-Simulink Converter3 : nesl_utility/PS-Simulink Converter  PhysicalDomain=network_engine_domain  SubClassName=ps_output  LeftPortType=input  RightPortType=output  PseudoPeriodic=off  Frequencies=[]  VectorFormat=1-D array  Unit=inherit  AffineConversion=off
  Prismatic OutFL : sm_lib/Joints/Prismatic Joint  JointMode=Normal  CompositeWrenchDir=FollowerOnBase  CompositeWrenchFrame=BaseFrame  SenseConstraintForce=off  SenseConstraintTorque=off  SenseTotalForce=off  SenseTotalTorque=off  PositionTargetSpecify=off  PositionTargetPriority=Low  PositionTargetValue=cylinders.ground.c1.pz0.sm  PositionTargetValueUnits=in  VelocityTargetSpecify=off  VelocityTargetPriority=High  VelocityTargetValue=0  VelocityTargetValueUnits=m/s  EquilibriumPosition=0  EquilibriumPositionUnits=m  SpringStiffness=0  SpringStiffnessUnits=N/m  DampingCoefficient=cylinders.ground.c1.b  DampingCoefficientUnits=N/(m/s)  LowerLimitSpecify=off  LowerLimitBound=-1  LowerLimitBoundUnits=m  LowerLimitStiffness=1e6  LowerLimitStiffnessUnits=N/m  LowerLimitDamping=1e3  LowerLimitDampingUnits=N/(m/s)  LowerLimitTransitionRegionWidth=1e-4  LowerLimitTransitionRegionWidthUnits=m  UpperLimitSpecify=off  UpperLimitBound=1  UpperLimitBoundUnits=m  UpperLimitStiffness=1e6  UpperLimitStiffnessUnits=N/m  UpperLimitDamping=1e3  UpperLimitDampingUnits=N/(m/s)  UpperLimitTransitionRegionWidth=1e-4  UpperLimitTransitionRegionWidthUnits=m  TorqueActuationMode=InputTorque  MotionActuationMode=ComputedMotion  SensePosition=on  SenseVelocity=on  SenseAcceleration=off  SenseTorqueForce=on  SenseLowerLimitTorqueForce=off  SenseUpperLimitTorqueForce=off
  Simscape Bus7 : SimscapeBus  HierarchyStrings=B;F
  Subsystem : Subsystem
  Subsystem1 : Subsystem
  BF : PMIOPort  Side=Right
  R : PMIOPort  Port=2  Side=Left
  m : Outport
  wires:
  PS-Simulink Converter1/1 -> Bus Creator1/1  "p"
  Bus Creator1/1 -> m/1  "OutFL"
  PS-Simulink Converter2/1 -> Bus Creator1/2  "v"
  PS-Simulink Converter3/1 -> Bus Creator1/3  "f"
  connections:
  Subsystem1/LConn1 -- Prismatic OutFL/RConn3 -- PS-Simulink Converter2/LConn1
  Ideal Force Sensor/LConn1 -- R/RConn1
  Subsystem/RConn1 -- Prismatic OutFL/LConn2
  PS-Simulink Converter1/LConn1 -- Prismatic OutFL/RConn2
  Ideal Translational Velocity Source/RConn1 -- Subsystem1/RConn1
  Simscape Bus7/LConn2 -- Prismatic OutFL/RConn1
  Simscape Bus7/LConn1 -- Prismatic OutFL/LConn1
  Simscape Bus7/RConn1 -- BF/RConn1
  Subsystem/LConn1 -- Ideal Force Sensor/RConn2
  Ideal Force Sensor/RConn1 -- Ideal Translational Velocity Source/LConn1
  Mechanical Translational Reference/LConn1 -- Ideal Translational Velocity Source/RConn2
  Prismatic OutFL/RConn4 -- PS-Simulink Converter3/LConn1

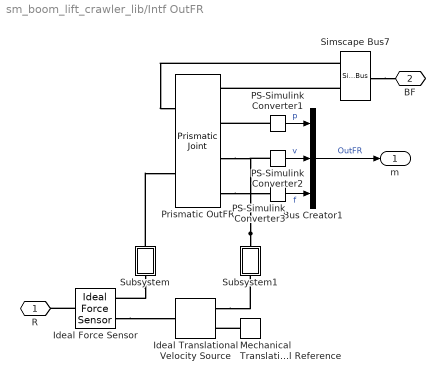
== system sm_boom_lift_crawler_lib/Intf OutFR ==
  Bus Creator1 : BusCreator  Inputs=3
  Ideal Force Sensor : fl_lib/Mechanical/Mechanical Sensors/Ideal Force Sensor
  Ideal Translational Velocity Source : fl_lib/Mechanical/Mechanical Sources/Ideal Translational Velocity Source
  Mechanical Translational Reference : fl_lib/Mechanical/Translational Elements/Mechanical Translational Reference
  PS-Simulink Converter1 : nesl_utility/PS-Simulink Converter  PhysicalDomain=network_engine_domain  SubClassName=ps_output  LeftPortType=input  RightPortType=output  PseudoPeriodic=off  Frequencies=[]  VectorFormat=1-D array  Unit=inherit  AffineConversion=off
  PS-Simulink Converter2 : nesl_utility/PS-Simulink Converter  PhysicalDomain=network_engine_domain  SubClassName=ps_output  LeftPortType=input  RightPortType=output  PseudoPeriodic=off  Frequencies=[]  VectorFormat=1-D array  Unit=inherit  AffineConversion=off
  PS-Simulink Converter3 : nesl_utility/PS-Simulink Converter  PhysicalDomain=network_engine_domain  SubClassName=ps_output  LeftPortType=input  RightPortType=output  PseudoPeriodic=off  Frequencies=[]  VectorFormat=1-D array  Unit=inherit  AffineConversion=off
  Prismatic OutFR : sm_lib/Joints/Prismatic Joint  JointMode=Normal  CompositeWrenchDir=FollowerOnBase  CompositeWrenchFrame=BaseFrame  SenseConstraintForce=off  SenseConstraintTorque=off  SenseTotalForce=off  SenseTotalTorque=off  PositionTargetSpecify=off  PositionTargetPriority=Low  PositionTargetValue=cylinders.ground.c2.pz0.sm  PositionTargetValueUnits=in  VelocityTargetSpecify=off  VelocityTargetPriority=High  VelocityTargetValue=0  VelocityTargetValueUnits=m/s  EquilibriumPosition=0  EquilibriumPositionUnits=m  SpringStiffness=0  SpringStiffnessUnits=N/m  DampingCoefficient=cylinders.ground.c1.b  DampingCoefficientUnits=N/(m/s)  LowerLimitSpecify=off  LowerLimitBound=-1  LowerLimitBoundUnits=m  LowerLimitStiffness=1e6  LowerLimitStiffnessUnits=N/m  LowerLimitDamping=1e3  LowerLimitDampingUnits=N/(m/s)  LowerLimitTransitionRegionWidth=1e-4  LowerLimitTransitionRegionWidthUnits=m  UpperLimitSpecify=off  UpperLimitBound=1  UpperLimitBoundUnits=m  UpperLimitStiffness=1e6  UpperLimitStiffnessUnits=N/m  UpperLimitDamping=1e3  UpperLimitDampingUnits=N/(m/s)  UpperLimitTransitionRegionWidth=1e-4  UpperLimitTransitionRegionWidthUnits=m  TorqueActuationMode=InputTorque  MotionActuationMode=ComputedMotion  SensePosition=on  SenseVelocity=on  SenseAcceleration=off  SenseTorqueForce=on  SenseLowerLimitTorqueForce=off  SenseUpperLimitTorqueForce=off
  Simscape Bus7 : SimscapeBus  HierarchyStrings=B;F
  Subsystem : Subsystem
  Subsystem1 : Subsystem
  R : PMIOPort  Side=Left
  BF : PMIOPort  Port=2  Side=Right
  m : Outport
  wires:
  PS-Simulink Converter1/1 -> Bus Creator1/1  "p"
  Bus Creator1/1 -> m/1  "OutFR"
  PS-Simulink Converter2/1 -> Bus Creator1/2  "v"
  PS-Simulink Converter3/1 -> Bus Creator1/3  "f"
  connections:
  Simscape Bus7/LConn1 -- Prismatic OutFR/LConn1
  Simscape Bus7/LConn2 -- Prismatic OutFR/RConn1
  Subsystem1/LConn1 -- Prismatic OutFR/RConn3 -- PS-Simulink Converter2/LConn1
  Simscape Bus7/RConn1 -- BF/RConn1
  Ideal Translational Velocity Source/RConn1 -- Subsystem1/RConn1
  Ideal Force Sensor/LConn1 -- R/RConn1
  PS-Simulink Converter1/LConn1 -- Prismatic OutFR/RConn2
  Subsystem/RConn1 -- Prismatic OutFR/LConn2
  Subsystem/LConn1 -- Ideal Force Sensor/RConn2
  Ideal Force Sensor/RConn1 -- Ideal Translational Velocity Source/LConn1
  Mechanical Translational Reference/LConn1 -- Ideal Translational Velocity Source/RConn2
  Prismatic OutFR/RConn4 -- PS-Simulink Converter3/LConn1
